simulink model "identifikalt_modell"  (R2024b)
settings: Solver=VariableStepAuto  StartTime=0.0  StopTime=20  RelTol=1e-3
values from neighbouring files (symbols this model uses):
  Ft1 = Phit1-Gtilde1*Ct1*Phit1    [ident_test.m]
  Ft2 = Phit2-Gtilde2*Ct2*Phit2    [ident_test.m]
  Gtilde1 = acker(Phit1',Phit1'*Ct1',[zoinf1 zoinf1 zoinf1 zoinf1]')'    [ident_test.m]
  Gtilde2 = acker(Phit2',Phit2'*Ct2',[zoinf2 zoinf2 zoinf2 zoinf2]')'    [ident_test.m]
  Ht1 = Gammat1-Gtilde1*Ct1*Gammat1    [ident_test.m]
  Ht2 = Gammat2-Gtilde2*Ct2*Gammat2    [ident_test.m]
  K1 = acker(Phi1,Gamma1,P1*0.935)    [ident_test.m]
  K2 = acker(Phi2,Gamma2,P2*0.949)    [ident_test.m]
  nl_x1 = sort(nlhw1.InputNonlinearity.BreakPoints(1,:))    [ident_test.m]
  nl_x2 = sort(nlhw2.InputNonlinearity.BreakPoints(1,:))    [ident_test.m]
  nl_y1 = sort(nlhw1.InputNonlinearity.BreakPoints(2,:))    [ident_test.m]
  nl_y2 = sort(nlhw2.InputNonlinearity.BreakPoints(2,:))    [ident_test.m]
  Nu1 = N1(4)    [ident_test.m]
  Nu2 = N2(4)    [ident_test.m]
  Nx1 = N1(1:3)    [ident_test.m]
  Nx2 = N2(1:3)    [ident_test.m]
undefined symbols (not defined in the file or in its folder): nlhw1, nlhw2
libraries: slident x2, simulink x1
settings Model: Creator=Asus  LastModifiedBy=Asus

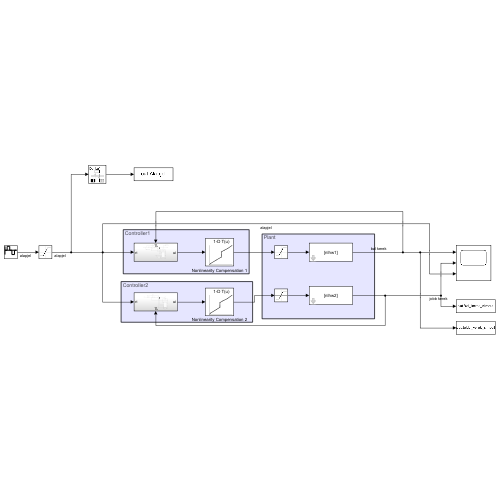
[thumbnail: Simulink's stored preview of the top-level diagram]
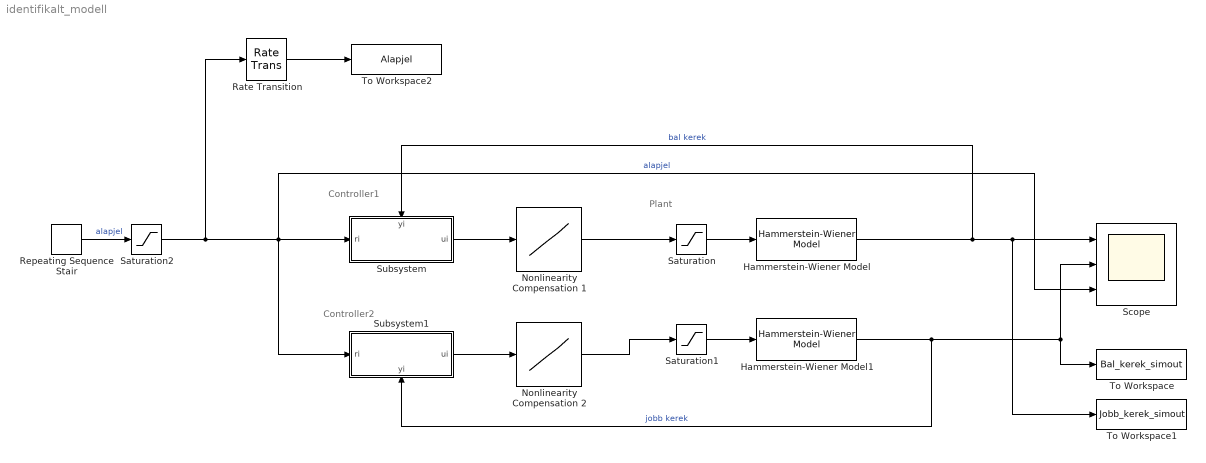
== system identifikalt_modell ==
  note: Controller2
  note: Controller1
  note: Plant
  Hammerstein-Wiener Model : slident/Models/Hammerstein-Wiener Model  sys=[nlhw1]  IC=Zero  X0i=0
  Hammerstein-Wiener Model1 : slident/Models/Hammerstein-Wiener Model  sys=[nlhw2]  IC=Zero  X0i=0
  Nonlinearity Compensation 1 : Lookup_n-D  NumberOfTableDimensions=1  BreakpointsForDimension1=nl_y1  Table=nl_x1  InternalRulePriority=Speed  RndMeth=Simplest
  Nonlinearity Compensation 2 : Lookup_n-D  NumberOfTableDimensions=1  BreakpointsForDimension1=nl_y2  Table=nl_x2  InternalRulePriority=Speed  RndMeth=Simplest
  Rate Transition : RateTransition  Deterministic=off  OutPortSampleTime=0.02
  Repeating Sequence Stair : simulink/Sources/Repeating Sequence Stair  OutValues=[0 0.5 0 -0.5 0].'  tsamp=5  OutMin=[]  OutMax=[]  OutDataTypeStr=double  OutputDataTypeScalingMode=double  OutDataType=fixdt(0,8)  ConRadixGroup=Best Precision: Vector-wise  OutScaling=2^-12
  Saturation : Saturate  UpperLimit=99  LowerLimit=-99
  Saturation1 : Saturate  UpperLimit=99  LowerLimit=-99
  Saturation2 : Saturate  UpperLimit=0.3  LowerLimit=-0.3
  Scope : Scope  NumInputPorts=3
  Subsystem : Subsystem
      settings: PortSchema="{\"entries\":[{\"content\":{\"sides\":[{\"content\":{\"connectorIds\":[\"In1\"]},\"type\":\"ConnectorPlacement.EquallySpacedRectSide\",\"uuid\":\"762af65c-5493-4531-a087-19dfb91d4669\"},{\"content\":{\"connectorIds\":[\"Out1\"],\"side\":\"RIGHT\"},\"type\":\"ConnectorPlacement.EquallySpacedRectSide\",\"uuid\":\"e7ca2abd-a113-4e6b-b577-39e76de0dcc0\"},{\"content\":{\"connectorIds\":[\"In2\"],\"side\":\"TOP\"},\"type\":\"ConnectorPlacement.EquallySpacedRectSide\",\"uuid\":\"a5b9fd54-bd54-4a71-a997-a97e3d12eca6\"}]},\"type\":\"ConnectorPlacement.EquallySpacedConnector\",\"uuid\":\"41852683-e60c-4889-8748-a112f36a566c\"}],\"packageUris\":[\"http://schema.mathworks.com/mf0/Connector/R2020b\"],\"version\":\"1.0\"}"
  Subsystem1 : Subsystem
      settings: PortSchema="{\"entries\":[{\"content\":{\"sides\":[{\"content\":{\"connectorIds\":[\"In1\"]},\"type\":\"ConnectorPlacement.EquallySpacedRectSide\",\"uuid\":\"762af65c-5493-4531-a087-19dfb91d4669\"},{\"content\":{\"connectorIds\":[\"Out1\"],\"side\":\"RIGHT\"},\"type\":\"ConnectorPlacement.EquallySpacedRectSide\",\"uuid\":\"e7ca2abd-a113-4e6b-b577-39e76de0dcc0\"},{\"content\":{\"side\":\"TOP\"},\"type\":\"ConnectorPlacement.EquallySpacedRectSide\",\"uuid\":\"a5b9fd54-bd54-4a71-a997-a97e3d12eca6\"},{\"content\":{\"connectorIds\":[\"In2\"],\"side\":\"BOTTOM\"},\"type\":\"ConnectorPlacement.EquallySpacedRectSide\",\"uuid\":\"b1d2a51b-d1f1-4dca-a82a-0eee8494887e\"}]},\"type\":\"ConnectorPlacement.EquallySpacedConnector\",\"uuid\":\"41852683-e60c-4889-8748-a112f36a566c\"}],\"packageUris\":[\"http://schema.mathworks.com/mf0/Connector/R2020b\"],\"version\":\"1.0\"}"
  To Workspace : ToWorkspace  VariableName=Bal_kerek_simout  SaveFormat=Timeseries  SampleTime=-1
  To Workspace1 : ToWorkspace  VariableName=Jobb_kerek_simout  SaveFormat=Timeseries  SampleTime=-1
  To Workspace2 : ToWorkspace  VariableName=Alapjel  SaveFormat=Timeseries  SampleTime=-1
  wires:
  Hammerstein-Wiener Model/1 -> Subsystem/2(yi), To Workspace1/1, Scope/1  "bal kerek"
  Hammerstein-Wiener Model1/1 -> To Workspace/1, Scope/2, Subsystem1/2(yi)  "jobb kerek"
  Nonlinearity Compensation 1/1 -> Saturation/1
  Nonlinearity Compensation 2/1 -> Saturation1/1
  Saturation/1 -> Hammerstein-Wiener Model/1
  Saturation1/1 -> Hammerstein-Wiener Model1/1
  Saturation2/1 -> Rate Transition/1, Scope/3, Subsystem1/1(ri), Subsystem/1(ri)  "alapjel"
  Subsystem/1(ui) -> Nonlinearity Compensation 1/1
  Subsystem1/1(ui) -> Nonlinearity Compensation 2/1
  Repeating Sequence Stair/1 -> Saturation2/1  "alapjel"
  Rate Transition/1 -> To Workspace2/1

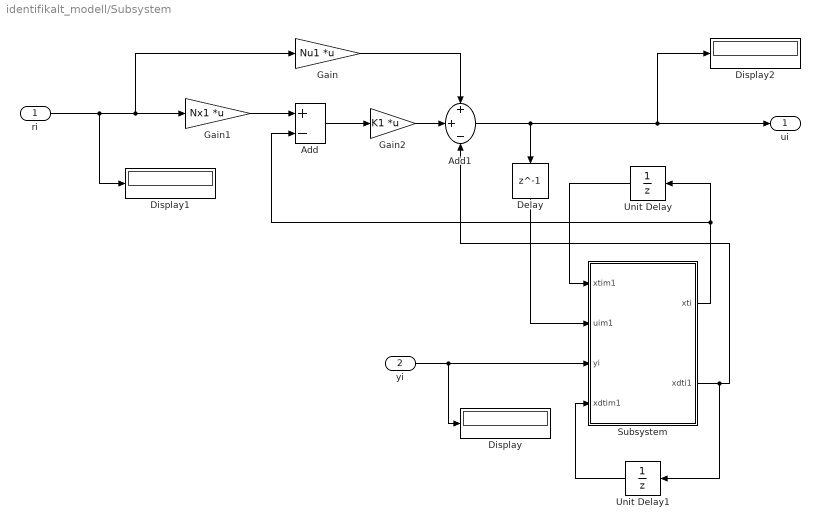
== system identifikalt_modell/Subsystem ==
  ri : Inport
  yi : Inport  Port=2
  Add : Sum  Inputs=+-
  Add1 : Sum  Inputs=++-
  Delay : Delay  DelayLength=1  InputProcessing=Columns as channels (frame based)
  Display : Display
  Display1 : Display
  Display2 : Display
  Gain : Gain  Gain=Nu1  Multiplication=Matrix(K*u)
  Gain1 : Gain  Gain=Nx1  Multiplication=Matrix(K*u)
  Gain2 : Gain  Gain=K1  Multiplication=Matrix(K*u)
  Subsystem : Subsystem
  Unit Delay : UnitDelay  SampleTime=-1  HasFrameUpgradeWarning=on
  Unit Delay1 : UnitDelay  SampleTime=-1  HasFrameUpgradeWarning=on
  ui : Outport
  wires:
  ri/1 -> Display1/1, Gain/1, Gain1/1
  Gain1/1 -> Add/1
  Gain/1 -> Add1/1
  Gain2/1 -> Add1/2
  Add/1 -> Gain2/1
  Add1/1 -> Delay/1, Display2/1, ui/1
  Delay/1 -> Subsystem/2(uim1)
  Subsystem/1(xti) -> Unit Delay/1, Add/2
  yi/1 -> Display/1, Subsystem/3(yi)
  Unit Delay/1 -> Subsystem/1(xtim1)
  Unit Delay1/1 -> Subsystem/4(xdtim1)
  Subsystem/2(xdti1) -> Unit Delay1/1, Add1/3

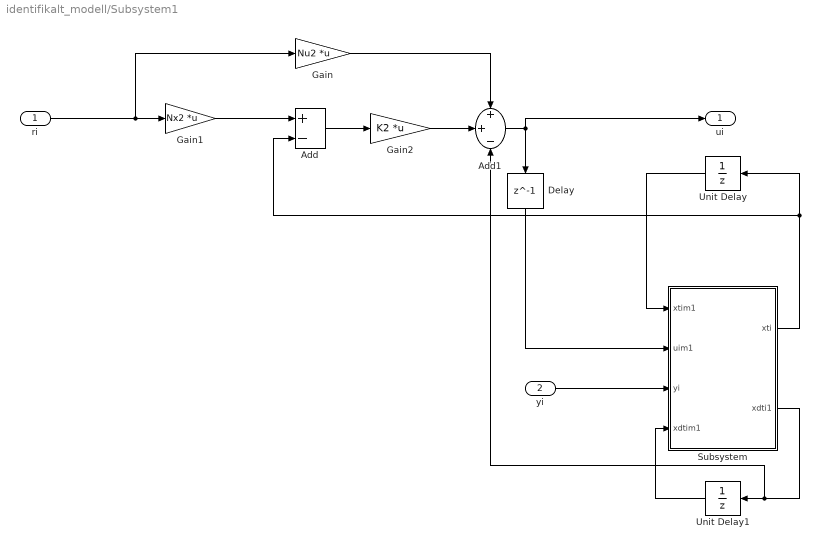
== system identifikalt_modell/Subsystem1 ==
  ri : Inport
  yi : Inport  Port=2
  Add : Sum  Inputs=+-
  Add1 : Sum  Inputs=++-
  Delay : Delay  DelayLength=1  InputProcessing=Columns as channels (frame based)
  Gain : Gain  Gain=Nu2  Multiplication=Matrix(K*u)
  Gain1 : Gain  Gain=Nx2  Multiplication=Matrix(K*u)
  Gain2 : Gain  Gain=K2  Multiplication=Matrix(K*u)
  Subsystem : Subsystem
  Unit Delay : UnitDelay  SampleTime=-1  HasFrameUpgradeWarning=on
  Unit Delay1 : UnitDelay  SampleTime=-1  HasFrameUpgradeWarning=on
  ui : Outport
  wires:
  ri/1 -> Gain/1, Gain1/1
  Gain1/1 -> Add/1
  Gain/1 -> Add1/1
  Gain2/1 -> Add1/2
  Add/1 -> Gain2/1
  Add1/1 -> ui/1, Delay/1
  Delay/1 -> Subsystem/2(uim1)
  Unit Delay/1 -> Subsystem/1(xtim1)
  Subsystem/1(xti) -> Add/2, Unit Delay/1
  yi/1 -> Subsystem/3(yi)
  Subsystem/2(xdti1) -> Add1/3, Unit Delay1/1
  Unit Delay1/1 -> Subsystem/4(xdtim1)

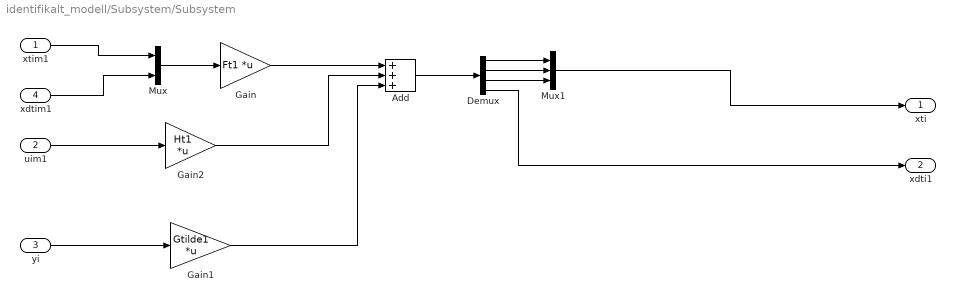
== system identifikalt_modell/Subsystem/Subsystem ==
  xtim1 : Inport
  uim1 : Inport  Port=2
  yi : Inport  Port=3
  xdtim1 : Inport  Port=4
  Add : Sum  Inputs=+++
  Demux : Demux
  Gain : Gain  Gain=Ft1  Multiplication=Matrix(K*u)
  Gain1 : Gain  Gain=Gtilde1  Multiplication=Matrix(K*u)
  Gain2 : Gain  Gain=Ht1  Multiplication=Matrix(K*u)
  Mux : Mux  Inputs=2
  Mux1 : Mux  Inputs=3
  xti : Outport
  xdti1 : Outport  Port=2
  wires:
  xdtim1/1 -> Mux/2
  xtim1/1 -> Mux/1
  Mux/1 -> Gain/1
  Gain/1 -> Add/1
  yi/1 -> Gain1/1
  uim1/1 -> Gain2/1
  Gain2/1 -> Add/2
  Gain1/1 -> Add/3
  Add/1 -> Demux/1
  Demux/1 -> Mux1/1
  Demux/2 -> Mux1/2
  Demux/3 -> Mux1/3
  Demux/4 -> xdti1/1
  Mux1/1 -> xti/1

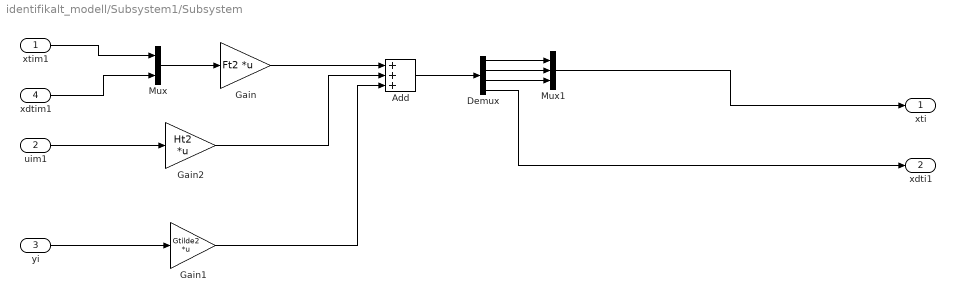
== system identifikalt_modell/Subsystem1/Subsystem ==
  xtim1 : Inport
  uim1 : Inport  Port=2
  yi : Inport  Port=3
  xdtim1 : Inport  Port=4
  Add : Sum  Inputs=+++
  Demux : Demux
  Gain : Gain  Gain=Ft2  Multiplication=Matrix(K*u)
  Gain1 : Gain  Gain=Gtilde2  Multiplication=Matrix(K*u)
  Gain2 : Gain  Gain=Ht2  Multiplication=Matrix(K*u)
  Mux : Mux  Inputs=2
  Mux1 : Mux  Inputs=3
  xti : Outport
  xdti1 : Outport  Port=2
  wires:
  xdtim1/1 -> Mux/2
  xtim1/1 -> Mux/1
  Mux/1 -> Gain/1
  Gain/1 -> Add/1
  yi/1 -> Gain1/1
  uim1/1 -> Gain2/1
  Gain2/1 -> Add/2
  Gain1/1 -> Add/3
  Add/1 -> Demux/1
  Demux/1 -> Mux1/1
  Demux/2 -> Mux1/2
  Demux/3 -> Mux1/3
  Demux/4 -> xdti1/1
  Mux1/1 -> xti/1
